simulink model "ukol_5_model"  (R2016a)
settings: Solver=VariableStepAuto  SolverMode=SingleTasking  StartTime=0.0  StopTime=1000  MaxStep=1e-2  RelTol=1e-3
undefined symbols (not defined in the file): A, B, C_1, D, k1, k1_2, k2, k2_2, kI, korekcni_zesileni
settings Model: Creator=tomas  LastModifiedBy=tomas
settings DebuggingCC: SFUnexpectedBacktrackingDiag=error  SFNoUnconditionalDefaultTransitionDiag=error
settings GRTTargetCC: TargetLangStandard=C99 (ISO)  GeneratePreprocessorConditionals=Use local settings
settings ConfigComp: CovMetricSettings=dwe  CovHtmlReporting=off  CovSaveCumulativeToWorkspaceVar=off  CovSaveSingleToWorkspaceVar=off  CovExternalEMLEnable=on

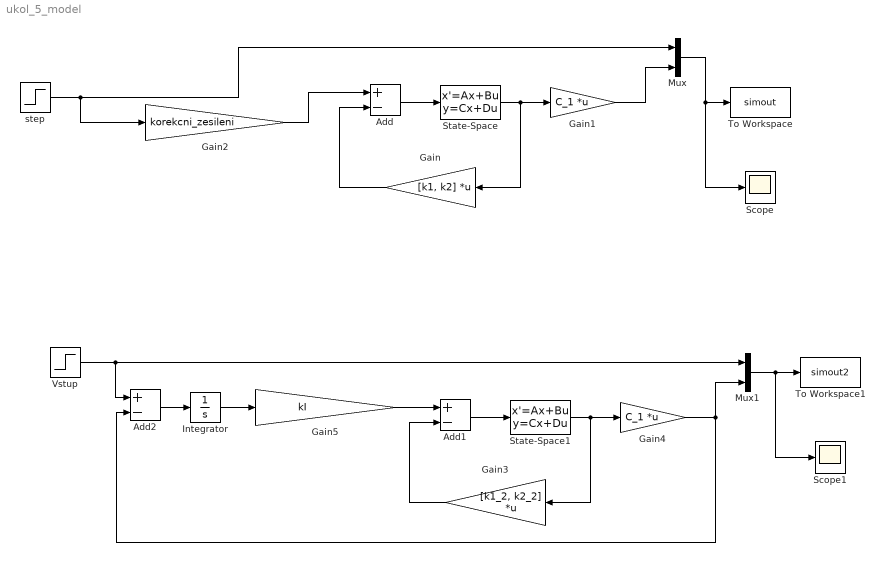
== system ukol_5_model ==
  Add : Sum  Inputs=+-
  Add1 : Sum  Inputs=+-
  Add2 : Sum  Inputs=+-
  Gain : Gain  Gain=[k1, k2]  Multiplication=Matrix(K*u)
  Gain1 : Gain  Gain=C_1  Multiplication=Matrix(K*u)
  Gain2 : Gain  Gain=korekcni_zesileni
  Gain3 : Gain  Gain=[k1_2, k2_2]  Multiplication=Matrix(K*u)
  Gain4 : Gain  Gain=C_1  Multiplication=Matrix(K*u)
  Gain5 : Gain  Gain=kI
  Integrator : Integrator
  Mux : Mux  Inputs=2
  Mux1 : Mux  Inputs=2
  Scope : Scope
  Scope1 : Scope
  State-Space : StateSpace  A=A  B=B  C=[1 0; 0 1]  D=D  X0=0
  State-Space1 : StateSpace  A=A  B=B  C=[1 0; 0 1]  D=D  X0=0
  To Workspace : ToWorkspace  VariableName=simout  SaveFormat=Timeseries  SampleTime=-1
  To Workspace1 : ToWorkspace  VariableName=simout2  SaveFormat=Timeseries  SampleTime=-1
  Vstup : Step  SampleTime=0
  step : Step  SampleTime=0
  wires:
  State-Space/1 -> Gain/1, Gain1/1
  Add/1 -> State-Space/1
  Gain/1 -> Add/2
  Gain1/1 -> Mux/2
  Mux/1 -> Scope/1, To Workspace/1
  step/1 -> Mux/1, Gain2/1
  Gain2/1 -> Add/1
  Gain5/1 -> Add1/1
  Gain4/1 -> Add2/2, Mux1/2
  State-Space1/1 -> Gain3/1, Gain4/1
  Add1/1 -> State-Space1/1
  Mux1/1 -> Scope1/1, To Workspace1/1
  Gain3/1 -> Add1/2
  Integrator/1 -> Gain5/1
  Add2/1 -> Integrator/1
  Vstup/1 -> Mux1/1, Add2/1
